simulink library "WECSim_Lib"  (R2014b)
settings: Solver=ode45  StartTime=0.0  StopTime=10.0  RelTol=1e-3
undefined symbols (not defined in the file): body, constraint, pto, simu, waves, X, Y, Z
libraries: nesl_utility x178, sm_lib x59, vrlib x12
(part 6 of 6)

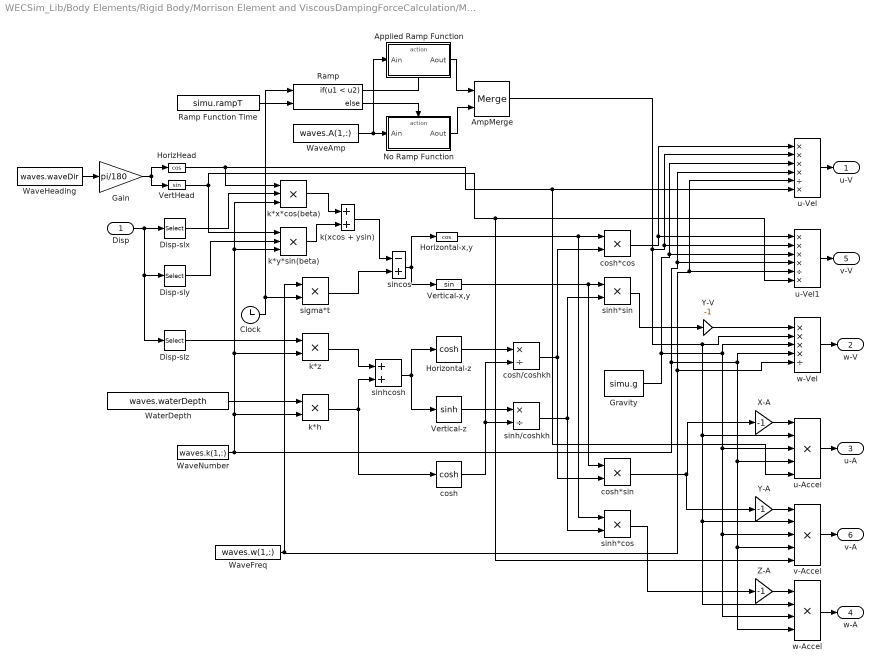
== system WECSim_Lib/Body Elements/Rigid Body/Morrison Element and ViscousDampingForceCalculation/Morrison Element Variant Subsystem/Morrison Element On/No Wave Excitation Force/MorrisonElements/OrbitalVelocity ==
  Disp : Inport
  AmpMerge : Merge
  Applied Ramp Function : Subsystem  TreatAsAtomicUnit=on
  Clock : Clock
  Disp-slx : Selector  InputPortWidth=3  Indices=[1]
  Disp-sly : Selector  InputPortWidth=3  Indices=[2]
  Disp-slz : Selector  InputPortWidth=3  Indices=[3]
  Gain : Gain  Gain=pi/180
  Gravity : Constant  Value=simu.g
  HorizHead : Trigonometry  Operator=cos
  Horizontal-x,y : Trigonometry  Operator=cos
  Horizontal-z : Trigonometry  Operator=cosh
  No Ramp Function : Subsystem  TreatAsAtomicUnit=on
  Ramp : If  NumInputs=2  IfExpression=u1 < u2
  Ramp Function Time : Constant  Value=simu.rampT
  VertHead : Trigonometry
  Vertical-x,y : Trigonometry
  Vertical-z : Trigonometry  Operator=sinh
  WaterDepth : Constant  Value=waves.waterDepth
  WaveAmp : Constant  Value=waves.A(1,:)
  WaveFreq : Constant  Value=waves.w(1,:)
  WaveHeading : Constant  Value=waves.waveDir
  WaveNumber : Constant  Value=waves.k(1,:)
  X-A : Gain  Gain=-1
  Y-A : Gain  Gain=-1
  Y-V : Gain  Gain=-1
  Z-A : Gain  Gain=-1
  cosh : Trigonometry  Operator=cosh
  cosh*cos : Product  Inputs=**
  cosh*sin : Product  Inputs=**
  cosh/coshkh : Product  Inputs=*/
  k(xcos + ysin) : Sum
  k*h : Product
  k*x*cos(beta) : Product  Inputs=3
  k*y*sin(beta) : Product  Inputs=3
  k*z : Product
  sigma*t : Product
  sincos : Sum  Inputs=-+
  sinh*cos : Product  Inputs=**
  sinh*sin : Product  Inputs=**
  sinh/coshkh : Product  Inputs=*/
  sinhcosh : Sum
  u-Accel : Product  Inputs=*****
  u-Vel : Product  Inputs=****/*
  u-Vel1 : Product  Inputs=****/*
  v-Accel : Product  Inputs=*****
  w-Accel : Product  Inputs=****
  w-Vel : Product  Inputs=****/
  u-V : Outport
  w-V : Outport  Port=2
  u-A : Outport  Port=3
  w-A : Outport  Port=4
  v-V : Outport  Port=5
  v-A : Outport  Port=6
  wires:
  Disp/1 -> Disp-slz/1, Disp-sly/1, Disp-slx/1
  WaveNumber/1 -> k*h/2, k*z/2, k*y*sin(beta)/3, k*x*cos(beta)/3, w-Vel/4, v-Accel/4, w-Accel/4, u-Accel/4, u-Vel1/4, u-Vel/4
  WaterDepth/1 -> k*h/1
  sigma*t/1 -> sincos/2
  sincos/1 -> Vertical-x,y/1, Horizontal-x,y/1
  k*z/1 -> sinhcosh/1
  k*h/1 -> cosh/1, sinhcosh/2
  sinhcosh/1 -> Vertical-z/1, Horizontal-z/1
  Horizontal-z/1 -> cosh/coshkh/1
  cosh/1 -> sinh/coshkh/2, cosh/coshkh/2
  Vertical-z/1 -> sinh/coshkh/1
  Vertical-x,y/1 -> cosh*sin/1, sinh*sin/1
  sinh/coshkh/1 -> sinh*cos/2, sinh*sin/2
  Horizontal-x,y/1 -> sinh*cos/1, cosh*cos/1
  cosh/coshkh/1 -> cosh*cos/2, cosh*sin/2
  Disp-sly/1 -> k*y*sin(beta)/2
  cosh*cos/1 -> u-Vel1/1, u-Vel/1
  AmpMerge/1 -> w-Vel/2, w-Accel/2, v-Accel/2, u-Accel/2, u-Vel1/2, u-Vel/2
  Gravity/1 -> w-Vel/3, v-Accel/3, w-Accel/3, u-Accel/3, u-Vel1/3, u-Vel/3
  sinh*sin/1 -> Y-V/1
  Y-V/1 -> w-Vel/1
  X-A/1 -> u-Accel/1
  Z-A/1 -> w-Accel/1
  w-Vel/1 -> w-V/1
  u-Accel/1 -> u-A/1
  w-Accel/1 -> w-A/1
  cosh*sin/1 -> Y-A/1, X-A/1
  sinh*cos/1 -> Z-A/1
  Ramp Function Time/1 -> Ramp/2
  Ramp/2 -> No Ramp Function/Action
  Ramp/1 -> Applied Ramp Function/Action
  Clock/1 -> Ramp/1, sigma*t/2
  No Ramp Function/1(Aout) -> AmpMerge/2
  Applied Ramp Function/1(Aout) -> AmpMerge/1
  Disp-slz/1 -> k*z/1
  WaveFreq/1 -> w-Vel/5, u-Vel1/5, u-Vel/5, sigma*t/1
  WaveAmp/1 -> Applied Ramp Function/1(Ain), No Ramp Function/1(Ain)
  WaveHeading/1 -> Gain/1
  Gain/1 -> HorizHead/1, VertHead/1
  Disp-slx/1 -> k*x*cos(beta)/2
  HorizHead/1 -> u-Accel/5, u-Vel/6, k*x*cos(beta)/1
  VertHead/1 -> k*y*sin(beta)/1, u-Vel1/6, v-Accel/5
  k*y*sin(beta)/1 -> k(xcos + ysin)/2
  k*x*cos(beta)/1 -> k(xcos + ysin)/1
  k(xcos + ysin)/1 -> sincos/1
  u-Vel1/1 -> v-V/1
  u-Vel/1 -> u-V/1
  Y-A/1 -> v-Accel/1
  v-Accel/1 -> v-A/1

== system WECSim_Lib/Body Elements/Rigid Body/Morrison Element and ViscousDampingForceCalculation/Morrison Element Variant Subsystem/Morrison Element On/No Wave Excitation Force/MorrisonElements/Rotation1 ==
  rot1 : Inport
  rot2 : Inport  Port=2
  rot3 : Inport  Port=3
  2 : Product
  3 : Product  Inputs=3
  7 : Product
  8 : Product  Inputs=3
  Combine : Concatenate  NumInputs=3  Mode=Multidimensional array  ConcatenateDimension=2
  Trigonometric Function{,1..2,6,9,11} (6 alike) : Trigonometry  Operator=cos
  Trigonometric Function{3..5,7..8,10} (6 alike) : Trigonometry
  rot11 : Product
  rot12 : Sum
  rot13 : Sum  Inputs=+-
  rot[1,1-3] : Outport
  wires:
  Trigonometric Function/1 -> rot11/1
  Trigonometric Function1/1 -> rot11/2
  rot11/1 -> Combine/1
  Trigonometric Function2/1 -> 2/1
  Trigonometric Function3/1 -> 2/2
  Trigonometric Function4/1 -> 3/1
  Trigonometric Function5/1 -> 3/2
  Trigonometric Function6/1 -> 3/3
  2/1 -> rot12/1
  3/1 -> rot12/2
  rot12/1 -> Combine/2
  Combine/1 -> rot[1,1-3]/1
  rot2/1 -> Trigonometric Function/1, Trigonometric Function5/1, Trigonometric Function10/1
  rot3/1 -> Trigonometric Function1/1, Trigonometric Function3/1, Trigonometric Function6/1, Trigonometric Function11/1, Trigonometric Function8/1
  rot1/1 -> Trigonometric Function2/1, Trigonometric Function4/1, Trigonometric Function9/1, Trigonometric Function7/1
  Trigonometric Function7/1 -> 7/1
  Trigonometric Function8/1 -> 7/2
  Trigonometric Function9/1 -> 8/1
  Trigonometric Function10/1 -> 8/2
  Trigonometric Function11/1 -> 8/3
  7/1 -> rot13/1
  8/1 -> rot13/2
  rot13/1 -> Combine/3

== system WECSim_Lib/Body Elements/Rigid Body/Morrison Element and ViscousDampingForceCalculation/Morrison Element Variant Subsystem/Morrison Element On/No Wave Excitation Force/MorrisonElements/Rotation2 ==
  rot1 : Inport
  rot2 : Inport  Port=2
  rot3 : Inport  Port=3
  2 : Product
  3 : Product  Inputs=3
  7 : Product
  8 : Product  Inputs=3
  Combine : Concatenate  NumInputs=3  Mode=Multidimensional array  ConcatenateDimension=2
  Gain : Gain  Gain=-1
  Trigonometric Function{,2..3,8..9} (5 alike) : Trigonometry  Operator=cos
  Trigonometric Function{1,4..7,10..11} (7 alike) : Trigonometry
  rot11 : Product
  rot12 : Sum  Inputs=+-
  rot13 : Sum
  rot[2,1-3] : Outport
  wires:
  Trigonometric Function/1 -> Gain/1
  Trigonometric Function1/1 -> rot11/2
  rot11/1 -> Combine/1
  Trigonometric Function2/1 -> 2/1
  Trigonometric Function3/1 -> 2/2
  Trigonometric Function4/1 -> 3/1
  Trigonometric Function5/1 -> 3/2
  Trigonometric Function6/1 -> 3/3
  2/1 -> rot12/1
  3/1 -> rot12/2
  rot12/1 -> Combine/2
  Combine/1 -> rot[2,1-3]/1
  rot2/1 -> Trigonometric Function/1, Trigonometric Function5/1, Trigonometric Function10/1
  rot3/1 -> Trigonometric Function1/1, Trigonometric Function3/1, Trigonometric Function6/1, Trigonometric Function11/1, Trigonometric Function8/1
  rot1/1 -> Trigonometric Function2/1, Trigonometric Function4/1, Trigonometric Function9/1, Trigonometric Function7/1
  Trigonometric Function7/1 -> 7/1
  Trigonometric Function8/1 -> 7/2
  Trigonometric Function9/1 -> 8/1
  Trigonometric Function10/1 -> 8/2
  Trigonometric Function11/1 -> 8/3
  7/1 -> rot13/1
  8/1 -> rot13/2
  rot13/1 -> Combine/3
  Gain/1 -> rot11/1

== system WECSim_Lib/Body Elements/Rigid Body/Morrison Element and ViscousDampingForceCalculation/Morrison Element Variant Subsystem/Morrison Element On/No Wave Excitation Force/MorrisonElements/Rotation3 ==
  rot1 : Inport
  rot2 : Inport  Port=2
  2 : Product
  7 : Product
  Combine : Concatenate  NumInputs=3  Mode=Multidimensional array  ConcatenateDimension=2
  Gain1 : Gain  Gain=-1
  TrigFun1 : Trigonometry
  TrigFun2 : Trigonometry
  TrigFun3 : Trigonometry  Operator=cos
  TrigFun4 : Trigonometry  Operator=cos
  TrigFun5 : Trigonometry  Operator=cos
  rot[3,1-3] : Outport
  wires:
  TrigFun1/1 -> Combine/1
  TrigFun3/1 -> 2/2
  2/1 -> Combine/2
  Combine/1 -> rot[3,1-3]/1
  rot2/1 -> TrigFun5/1, TrigFun3/1, TrigFun1/1
  TrigFun4/1 -> 7/1
  TrigFun5/1 -> 7/2
  rot1/1 -> TrigFun2/1, TrigFun4/1
  7/1 -> Combine/3
  TrigFun2/1 -> Gain1/1
  Gain1/1 -> 2/1

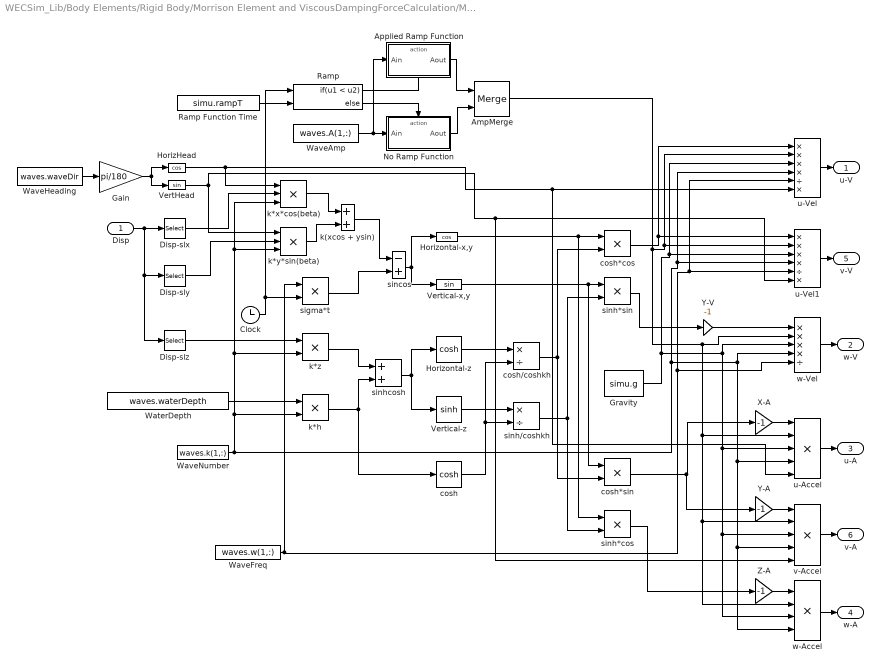
== system WECSim_Lib/Body Elements/Rigid Body/Morrison Element and ViscousDampingForceCalculation/Morrison Element Variant Subsystem/Morrison Element On/Regular Wave Excitation Force/MorrisonElements/OrbitalVelocity ==
  Disp : Inport
  AmpMerge : Merge
  Applied Ramp Function : Subsystem  TreatAsAtomicUnit=on
  Clock : Clock
  Disp-slx : Selector  InputPortWidth=3  Indices=[1]
  Disp-sly : Selector  InputPortWidth=3  Indices=[2]
  Disp-slz : Selector  InputPortWidth=3  Indices=[3]
  Gain : Gain  Gain=pi/180
  Gravity : Constant  Value=simu.g
  HorizHead : Trigonometry  Operator=cos
  Horizontal-x,y : Trigonometry  Operator=cos
  Horizontal-z : Trigonometry  Operator=cosh
  No Ramp Function : Subsystem  TreatAsAtomicUnit=on
  Ramp : If  NumInputs=2  IfExpression=u1 < u2
  Ramp Function Time : Constant  Value=simu.rampT
  VertHead : Trigonometry
  Vertical-x,y : Trigonometry
  Vertical-z : Trigonometry  Operator=sinh
  WaterDepth : Constant  Value=waves.waterDepth
  WaveAmp : Constant  Value=waves.A(1,:)
  WaveFreq : Constant  Value=waves.w(1,:)
  WaveHeading : Constant  Value=waves.waveDir
  WaveNumber : Constant  Value=waves.k(1,:)
  X-A : Gain  Gain=-1
  Y-A : Gain  Gain=-1
  Y-V : Gain  Gain=-1
  Z-A : Gain  Gain=-1
  cosh : Trigonometry  Operator=cosh
  cosh*cos : Product  Inputs=**
  cosh*sin : Product  Inputs=**
  cosh/coshkh : Product  Inputs=*/
  k(xcos + ysin) : Sum
  k*h : Product
  k*x*cos(beta) : Product  Inputs=3
  k*y*sin(beta) : Product  Inputs=3
  k*z : Product
  sigma*t : Product
  sincos : Sum  Inputs=-+
  sinh*cos : Product  Inputs=**
  sinh*sin : Product  Inputs=**
  sinh/coshkh : Product  Inputs=*/
  sinhcosh : Sum
  u-Accel : Product  Inputs=*****
  u-Vel : Product  Inputs=****/*
  u-Vel1 : Product  Inputs=****/*
  v-Accel : Product  Inputs=*****
  w-Accel : Product  Inputs=****
  w-Vel : Product  Inputs=****/
  u-V : Outport
  w-V : Outport  Port=2
  u-A : Outport  Port=3
  w-A : Outport  Port=4
  v-V : Outport  Port=5
  v-A : Outport  Port=6
  wires:
  Disp/1 -> Disp-slz/1, Disp-sly/1, Disp-slx/1
  WaveNumber/1 -> k*h/2, k*z/2, k*y*sin(beta)/3, k*x*cos(beta)/3, w-Vel/4, v-Accel/4, w-Accel/4, u-Accel/4, u-Vel1/4, u-Vel/4
  WaterDepth/1 -> k*h/1
  sigma*t/1 -> sincos/2
  sincos/1 -> Vertical-x,y/1, Horizontal-x,y/1
  k*z/1 -> sinhcosh/1
  k*h/1 -> cosh/1, sinhcosh/2
  sinhcosh/1 -> Vertical-z/1, Horizontal-z/1
  Horizontal-z/1 -> cosh/coshkh/1
  cosh/1 -> sinh/coshkh/2, cosh/coshkh/2
  Vertical-z/1 -> sinh/coshkh/1
  Vertical-x,y/1 -> cosh*sin/1, sinh*sin/1
  sinh/coshkh/1 -> sinh*cos/2, sinh*sin/2
  Horizontal-x,y/1 -> sinh*cos/1, cosh*cos/1
  cosh/coshkh/1 -> cosh*cos/2, cosh*sin/2
  Disp-sly/1 -> k*y*sin(beta)/2
  cosh*cos/1 -> u-Vel1/1, u-Vel/1
  AmpMerge/1 -> w-Vel/2, w-Accel/2, v-Accel/2, u-Accel/2, u-Vel1/2, u-Vel/2
  Gravity/1 -> w-Vel/3, v-Accel/3, w-Accel/3, u-Accel/3, u-Vel1/3, u-Vel/3
  sinh*sin/1 -> Y-V/1
  Y-V/1 -> w-Vel/1
  X-A/1 -> u-Accel/1
  Z-A/1 -> w-Accel/1
  w-Vel/1 -> w-V/1
  u-Accel/1 -> u-A/1
  w-Accel/1 -> w-A/1
  cosh*sin/1 -> Y-A/1, X-A/1
  sinh*cos/1 -> Z-A/1
  Ramp Function Time/1 -> Ramp/2
  Ramp/2 -> No Ramp Function/Action
  Ramp/1 -> Applied Ramp Function/Action
  Clock/1 -> Ramp/1, sigma*t/2
  No Ramp Function/1(Aout) -> AmpMerge/2
  Applied Ramp Function/1(Aout) -> AmpMerge/1
  Disp-slz/1 -> k*z/1
  WaveFreq/1 -> w-Vel/5, u-Vel1/5, u-Vel/5, sigma*t/1
  WaveAmp/1 -> Applied Ramp Function/1(Ain), No Ramp Function/1(Ain)
  WaveHeading/1 -> Gain/1
  Gain/1 -> HorizHead/1, VertHead/1
  Disp-slx/1 -> k*x*cos(beta)/2
  HorizHead/1 -> u-Accel/5, u-Vel/6, k*x*cos(beta)/1
  VertHead/1 -> k*y*sin(beta)/1, u-Vel1/6, v-Accel/5
  k*y*sin(beta)/1 -> k(xcos + ysin)/2
  k*x*cos(beta)/1 -> k(xcos + ysin)/1
  k(xcos + ysin)/1 -> sincos/1
  u-Vel1/1 -> v-V/1
  u-Vel/1 -> u-V/1
  Y-A/1 -> v-Accel/1
  v-Accel/1 -> v-A/1

== system WECSim_Lib/Body Elements/Rigid Body/Morrison Element and ViscousDampingForceCalculation/Morrison Element Variant Subsystem/Morrison Element On/Regular Wave Excitation Force/MorrisonElements/Rotation1 ==
  rot1 : Inport
  rot2 : Inport  Port=2
  rot3 : Inport  Port=3
  2 : Product
  3 : Product  Inputs=3
  7 : Product
  8 : Product  Inputs=3
  Combine : Concatenate  NumInputs=3  Mode=Multidimensional array  ConcatenateDimension=2
  Trigonometric Function{,1..2,6,9,11} (6 alike) : Trigonometry  Operator=cos
  Trigonometric Function{3..5,7..8,10} (6 alike) : Trigonometry
  rot11 : Product
  rot12 : Sum
  rot13 : Sum  Inputs=+-
  rot[1,1-3] : Outport
  wires:
  Trigonometric Function/1 -> rot11/1
  Trigonometric Function1/1 -> rot11/2
  rot11/1 -> Combine/1
  Trigonometric Function2/1 -> 2/1
  Trigonometric Function3/1 -> 2/2
  Trigonometric Function4/1 -> 3/1
  Trigonometric Function5/1 -> 3/2
  Trigonometric Function6/1 -> 3/3
  2/1 -> rot12/1
  3/1 -> rot12/2
  rot12/1 -> Combine/2
  Combine/1 -> rot[1,1-3]/1
  rot2/1 -> Trigonometric Function/1, Trigonometric Function5/1, Trigonometric Function10/1
  rot3/1 -> Trigonometric Function1/1, Trigonometric Function3/1, Trigonometric Function6/1, Trigonometric Function11/1, Trigonometric Function8/1
  rot1/1 -> Trigonometric Function2/1, Trigonometric Function4/1, Trigonometric Function9/1, Trigonometric Function7/1
  Trigonometric Function7/1 -> 7/1
  Trigonometric Function8/1 -> 7/2
  Trigonometric Function9/1 -> 8/1
  Trigonometric Function10/1 -> 8/2
  Trigonometric Function11/1 -> 8/3
  7/1 -> rot13/1
  8/1 -> rot13/2
  rot13/1 -> Combine/3

== system WECSim_Lib/Body Elements/Rigid Body/Morrison Element and ViscousDampingForceCalculation/Morrison Element Variant Subsystem/Morrison Element On/Regular Wave Excitation Force/MorrisonElements/Rotation2 ==
  rot1 : Inport
  rot2 : Inport  Port=2
  rot3 : Inport  Port=3
  2 : Product
  3 : Product  Inputs=3
  7 : Product
  8 : Product  Inputs=3
  Combine : Concatenate  NumInputs=3  Mode=Multidimensional array  ConcatenateDimension=2
  Gain : Gain  Gain=-1
  Trigonometric Function{,2..3,8..9} (5 alike) : Trigonometry  Operator=cos
  Trigonometric Function{1,4..7,10..11} (7 alike) : Trigonometry
  rot11 : Product
  rot12 : Sum  Inputs=+-
  rot13 : Sum
  rot[2,1-3] : Outport
  wires:
  Trigonometric Function/1 -> Gain/1
  Trigonometric Function1/1 -> rot11/2
  rot11/1 -> Combine/1
  Trigonometric Function2/1 -> 2/1
  Trigonometric Function3/1 -> 2/2
  Trigonometric Function4/1 -> 3/1
  Trigonometric Function5/1 -> 3/2
  Trigonometric Function6/1 -> 3/3
  2/1 -> rot12/1
  3/1 -> rot12/2
  rot12/1 -> Combine/2
  Combine/1 -> rot[2,1-3]/1
  rot2/1 -> Trigonometric Function/1, Trigonometric Function5/1, Trigonometric Function10/1
  rot3/1 -> Trigonometric Function1/1, Trigonometric Function3/1, Trigonometric Function6/1, Trigonometric Function11/1, Trigonometric Function8/1
  rot1/1 -> Trigonometric Function2/1, Trigonometric Function4/1, Trigonometric Function9/1, Trigonometric Function7/1
  Trigonometric Function7/1 -> 7/1
  Trigonometric Function8/1 -> 7/2
  Trigonometric Function9/1 -> 8/1
  Trigonometric Function10/1 -> 8/2
  Trigonometric Function11/1 -> 8/3
  7/1 -> rot13/1
  8/1 -> rot13/2
  rot13/1 -> Combine/3
  Gain/1 -> rot11/1

== system WECSim_Lib/Body Elements/Rigid Body/Morrison Element and ViscousDampingForceCalculation/Morrison Element Variant Subsystem/Morrison Element On/Regular Wave Excitation Force/MorrisonElements/Rotation3 ==
  rot1 : Inport
  rot2 : Inport  Port=2
  2 : Product
  7 : Product
  Combine : Concatenate  NumInputs=3  Mode=Multidimensional array  ConcatenateDimension=2
  Gain1 : Gain  Gain=-1
  TrigFun1 : Trigonometry
  TrigFun2 : Trigonometry
  TrigFun3 : Trigonometry  Operator=cos
  TrigFun4 : Trigonometry  Operator=cos
  TrigFun5 : Trigonometry  Operator=cos
  rot[3,1-3] : Outport
  wires:
  TrigFun1/1 -> Combine/1
  TrigFun3/1 -> 2/2
  2/1 -> Combine/2
  Combine/1 -> rot[3,1-3]/1
  rot2/1 -> TrigFun5/1, TrigFun3/1, TrigFun1/1
  TrigFun4/1 -> 7/1
  TrigFun5/1 -> 7/2
  rot1/1 -> TrigFun2/1, TrigFun4/1
  7/1 -> Combine/3
  TrigFun2/1 -> Gain1/1
  Gain1/1 -> 2/1

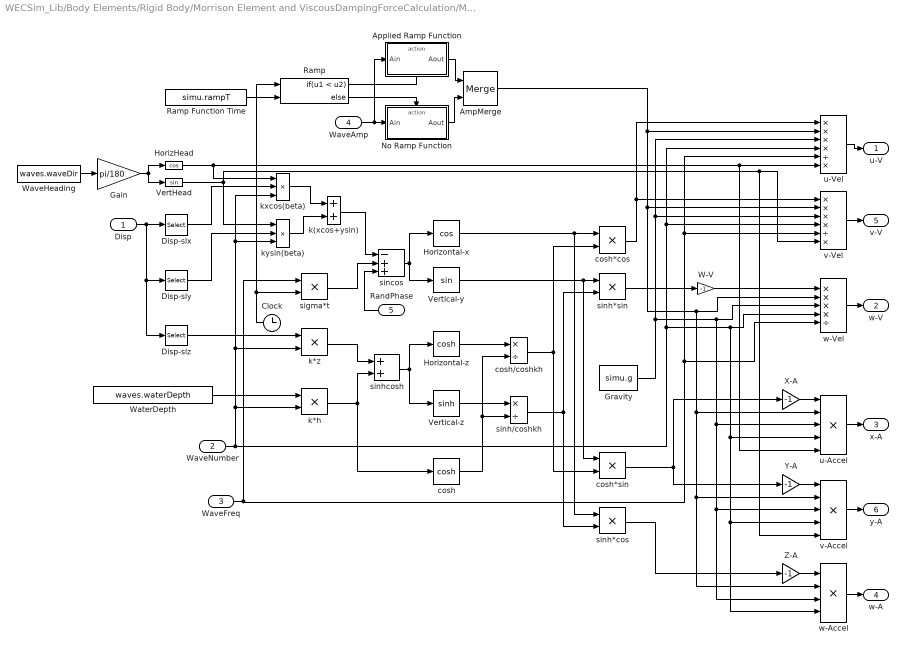
== system WECSim_Lib/Body Elements/Rigid Body/Morrison Element and ViscousDampingForceCalculation/Morrison Element Variant Subsystem/Morrison Element On/Irregular Wave Excitation Force/MorrisonElements/MorisonElementIrregular/OrbitalVelocity ==
  Disp : Inport
  WaveNumber : Inport  Port=2
  WaveFreq : Inport  Port=3
  WaveAmp : Inport  Port=4
  RandPhase : Inport  Port=5
  AmpMerge : Merge
  Applied Ramp Function : Subsystem  TreatAsAtomicUnit=on
  Clock : Clock
  Disp-slx : Selector  InputPortWidth=3  Indices=[1]
  Disp-sly : Selector  InputPortWidth=3  Indices=[2]
  Disp-slz : Selector  InputPortWidth=3  Indices=[3]
  Gain : Gain  Gain=pi/180
  Gravity : Constant  Value=simu.g
  HorizHead : Trigonometry  Operator=cos
  Horizontal-x : Trigonometry  Operator=cos
  Horizontal-z : Trigonometry  Operator=cosh
  No Ramp Function : Subsystem  TreatAsAtomicUnit=on
  Ramp : If  NumInputs=2  IfExpression=u1 < u2
  Ramp Function Time : Constant  Value=simu.rampT
  VertHead : Trigonometry
  Vertical-y : Trigonometry
  Vertical-z : Trigonometry  Operator=sinh
  W-V : Gain  Gain=-1
  WaterDepth : Constant  Value=waves.waterDepth
  WaveHeading : Constant  Value=waves.waveDir
  X-A : Gain  Gain=-1
  Y-A : Gain  Gain=-1
  Z-A : Gain  Gain=-1
  cosh : Trigonometry  Operator=cosh
  cosh*cos : Product  Inputs=**
  cosh*sin : Product  Inputs=**
  cosh/coshkh : Product  Inputs=*/
  k(xcos+ysin) : Sum
  k*h : Product
  k*z : Product
  kxcos(beta) : Product  Inputs=3
  kysin(beta) : Product  Inputs=3
  sigma*t : Product
  sincos : Sum  Inputs=-++
  sinh*cos : Product  Inputs=**
  sinh*sin : Product  Inputs=**
  sinh/coshkh : Product  Inputs=*/
  sinhcosh : Sum
  u-Accel : Product  Inputs=*****
  u-Vel : Product  Inputs=****/*
  v-Accel : Product  Inputs=*****
  v-Vel : Product  Inputs=****/*
  w-Accel : Product  Inputs=****
  w-Vel : Product  Inputs=****/
  u-V : Outport
  w-V : Outport  Port=2
  x-A : Outport  Port=3
  w-A : Outport  Port=4
  v-V : Outport  Port=5
  y-A : Outport  Port=6
  wires:
  Disp/1 -> Disp-slz/1, Disp-sly/1, Disp-slx/1
  WaveNumber/1 -> w-Vel/4, v-Accel/4, w-Accel/4, u-Accel/4, u-Vel/4, v-Vel/4, k*h/2, k*z/2, kysin(beta)/3, kxcos(beta)/3
  WaveFreq/1 -> sigma*t/1, u-Vel/5, v-Vel/5, w-Vel/5
  WaterDepth/1 -> k*h/1
  sigma*t/1 -> sincos/2
  sincos/1 -> Vertical-y/1, Horizontal-x/1
  k*z/1 -> sinhcosh/1
  k*h/1 -> cosh/1, sinhcosh/2
  sinhcosh/1 -> Vertical-z/1, Horizontal-z/1
  Horizontal-z/1 -> cosh/coshkh/1
  cosh/1 -> sinh/coshkh/2, cosh/coshkh/2
  Vertical-z/1 -> sinh/coshkh/1
  Vertical-y/1 -> sinh*sin/1, cosh*sin/1
  sinh/coshkh/1 -> sinh*cos/2, sinh*sin/2
  Horizontal-x/1 -> cosh*cos/1, sinh*cos/1
  cosh/coshkh/1 -> cosh*cos/2, cosh*sin/2
  Disp-sly/1 -> kysin(beta)/2
  cosh*cos/1 -> u-Vel/1, v-Vel/1
  AmpMerge/1 -> w-Vel/2, w-Accel/2, v-Accel/2, u-Accel/2, v-Vel/2, u-Vel/2
  sinh*sin/1 -> W-V/1
  W-V/1 -> w-Vel/1
  X-A/1 -> u-Accel/1
  Z-A/1 -> w-Accel/1
  u-Vel/1 -> u-V/1
  w-Vel/1 -> w-V/1
  u-Accel/1 -> x-A/1
  w-Accel/1 -> w-A/1
  cosh*sin/1 -> Y-A/1, X-A/1
  sinh*cos/1 -> Z-A/1
  Ramp Function Time/1 -> Ramp/2
  Ramp/2 -> No Ramp Function/Action
  Ramp/1 -> Applied Ramp Function/Action
  Clock/1 -> sigma*t/2, Ramp/1
  WaveAmp/1 -> Applied Ramp Function/1(Ain), No Ramp Function/1(Ain)
  No Ramp Function/1(Aout) -> AmpMerge/2
  Applied Ramp Function/1(Aout) -> AmpMerge/1
  Disp-slz/1 -> k*z/1
  RandPhase/1 -> sincos/3
  WaveHeading/1 -> Gain/1
  Gain/1 -> HorizHead/1, VertHead/1
  Disp-slx/1 -> kxcos(beta)/2
  HorizHead/1 -> kxcos(beta)/1, u-Vel/6, u-Accel/5
  VertHead/1 -> kysin(beta)/1, v-Accel/5, v-Vel/6
  kysin(beta)/1 -> k(xcos+ysin)/2
  kxcos(beta)/1 -> k(xcos+ysin)/1
  k(xcos+ysin)/1 -> sincos/1
  v-Vel/1 -> v-V/1
  Gravity/1 -> w-Vel/3, v-Accel/3, w-Accel/3, u-Accel/3, u-Vel/3, v-Vel/3
  Y-A/1 -> v-Accel/1
  v-Accel/1 -> y-A/1

== system WECSim_Lib/Body Elements/Rigid Body/Morrison Element and ViscousDampingForceCalculation/Morrison Element Variant Subsystem/Morrison Element On/No Wave Excitation Force/MorrisonElements/OrbitalVelocity/Applied Ramp Function ==
  Ain : Inport
  Action Port : ActionPort
  Add : Sum
  Constant : Constant  Value=2
  Constant1 : Constant
  Divide : Product  Inputs=**/
  Sine Wave : Sin  Frequency=pi/simu.rampT  Phase=pi+pi/2  SampleTime=0
  Aout : Outport
  wires:
  Ain/1 -> Divide/1
  Divide/1 -> Aout/1
  Constant/1 -> Divide/3
  Constant1/1 -> Add/1
  Sine Wave/1 -> Add/2
  Add/1 -> Divide/2

== system WECSim_Lib/Body Elements/Rigid Body/Morrison Element and ViscousDampingForceCalculation/Morrison Element Variant Subsystem/Morrison Element On/No Wave Excitation Force/MorrisonElements/OrbitalVelocity/No Ramp Function ==
  Ain : Inport
  Action Port : ActionPort
  Aout : Outport
  wires:
  Ain/1 -> Aout/1

== system WECSim_Lib/Body Elements/Rigid Body/Morrison Element and ViscousDampingForceCalculation/Morrison Element Variant Subsystem/Morrison Element On/Regular Wave Excitation Force/MorrisonElements/OrbitalVelocity/Applied Ramp Function ==
  Ain : Inport
  Action Port : ActionPort
  Add : Sum
  Constant : Constant  Value=2
  Constant1 : Constant
  Divide : Product  Inputs=**/
  Sine Wave : Sin  Frequency=pi/simu.rampT  Phase=pi+pi/2  SampleTime=0
  Aout : Outport
  wires:
  Ain/1 -> Divide/1
  Divide/1 -> Aout/1
  Constant/1 -> Divide/3
  Constant1/1 -> Add/1
  Sine Wave/1 -> Add/2
  Add/1 -> Divide/2

== system WECSim_Lib/Body Elements/Rigid Body/Morrison Element and ViscousDampingForceCalculation/Morrison Element Variant Subsystem/Morrison Element On/Regular Wave Excitation Force/MorrisonElements/OrbitalVelocity/No Ramp Function ==
  Ain : Inport
  Action Port : ActionPort
  Aout : Outport
  wires:
  Ain/1 -> Aout/1

== system WECSim_Lib/Body Elements/Rigid Body/Morrison Element and ViscousDampingForceCalculation/Morrison Element Variant Subsystem/Morrison Element On/Irregular Wave Excitation Force/MorrisonElements/MorisonElementIrregular/OrbitalVelocity/Applied Ramp Function ==
  Ain : Inport
  Action Port : ActionPort
  Add : Sum
  Constant : Constant  Value=2
  Constant1 : Constant
  Divide : Product  Inputs=**/
  Sine Wave : Sin  Frequency=pi/simu.rampT  Phase=pi+pi/2  SampleTime=0
  Aout : Outport
  wires:
  Ain/1 -> Divide/1
  Divide/1 -> Aout/1
  Constant/1 -> Divide/3
  Constant1/1 -> Add/1
  Sine Wave/1 -> Add/2
  Add/1 -> Divide/2

== system WECSim_Lib/Body Elements/Rigid Body/Morrison Element and ViscousDampingForceCalculation/Morrison Element Variant Subsystem/Morrison Element On/Irregular Wave Excitation Force/MorrisonElements/MorisonElementIrregular/OrbitalVelocity/No Ramp Function ==
  Ain : Inport
  Action Port : ActionPort
  Aout : Outport
  wires:
  Ain/1 -> Aout/1

== matlab function WECSim_Lib/Body Elements/Rigid Body/Wave Diffraction and Excitation Force Calculation/Nonlinear FK Force Variant Subsystem/With Nonlinear FroudeKrylov Force/Diffraction and Excitation Forces ==
  data: x input; elv input; center input; f output; tnorm input; area input; rho input; g input; cg input; AH input; w input; dw input; wDepth input; deepWaterWave input; k input; typeNum input; t input; phaseRand input; wp output; wpMeanFS output; dt input; dtFe input
function [f, wp, wpMeanFS]  = nonFKForce(x,elv,center,tnorm,area,rho,g,cg,AH,w,dw,wDepth,deepWaterWave,k,typeNum,t,phaseRand, dt, dtFe)
% Function to calculate buoyancy force and moment on a triangulated surface
% NOTE: This function assumes that the STL file is imported with its CG at 0,0,0

% Logic to calculate nonFKForce at reduced sample time
persistent oldForce
persistent oldWp
persistent oldWpMeanFs

if isempty(oldForce)
    [f, wp, wpMeanFS] = calc_force(x,elv,center,tnorm,area,rho,g,cg,AH,w,dw,wDepth,deepWaterWave,k,typeNum,t,phaseRand);
    oldForce = f;
    oldWp = wp;
    oldWpMeanFs = wpMeanFS;
else
    if mod(t, dtFe) < dt/2
        [f, wp, wpMeanFS] = calc_force(x,elv,center,tnorm,area,rho,g,cg,AH,w,dw,wDepth,deepWaterWave,k,typeNum,t,phaseRand);
        oldForce = f;
        oldWp = wp;
        oldWpMeanFs = wpMeanFS;
    else
        f = oldForce;
        wp = oldWp;
        wpMeanFS = oldWpMeanFs;
    end
end
end

function [f, wp, wpMeanFS]  = calc_force(x,elv,center,tnorm,area,rho,g,cg,AH,w,dw,wDepth,deepWaterWave,k,typeNum,t,phaseRand)
% Compute new tri coords after cog rotation and translation
centerMeanFS = offsetXYZ(center,cg);
avMeanFS     = tnorm .* [area area area];

% Compute new tri coords after cog rotation and translation
center = rotateXYZ(center,[1 0 0],x(4));
center = rotateXYZ(center,[0 1 0],x(5));
center = rotateXYZ(center,[0 0 1],x(6));
center = offsetXYZ(center,x);
center = offsetXYZ(center,cg);
% Compute new normal vectors coords after cog rotation and translation
tnorm = rotateXYZ(tnorm,[1 0 0],x(4));
tnorm = rotateXYZ(tnorm,[0 1 0],x(5));
tnorm = rotateXYZ(tnorm,[0 0 1],x(6));

% Copute area vectors
av = tnorm .* [area area area];

% Calculate the free surface
wpMeanFS=pDis(centerMeanFS,       0,AH,w,dw,wDepth,deepWaterWave,t,k,phaseRand,typeNum,rho,g);
wp      =pDis(center      ,     elv,AH,w,dw,wDepth,deepWaterWave,t,k,phaseRand,typeNum,rho,g);

% Calculate the hydrostatic forces
f_linear   =FK(centerMeanFS,       cg,avMeanFS,wpMeanFS);
f_nonLinear=FK(center      ,x(1:3)+cg,av      ,wp      ); 
f = f_nonLinear-f_linear;
end

function verts = offsetXYZ(verts,x)
% Function to move the position vertices
verts(:,1) = verts(:,1) + x(1);
verts(:,2) = verts(:,2) + x(2);
verts(:,3) = verts(:,3) + x(3);
end

function xn = rotateXYZ(x,ax,t)
	% function to rotate a point about an arbitrary axis
	% x: 3-componenet coordiantes
	% ax: axis about which to rotate (must be a normal vector)
	% t: rotation angle
	% xn: new coordinates after rotation
	rotMat = zeros(3);
	rotMat(1,1) = ax(1)*ax(1)*(1-cos(t))    + cos(t);
	rotMat(1,2) = ax(2)*ax(1)*(1-cos(t))    + ax(3)*sin(t);
	rotMat(1,3) = ax(3)*ax(1)*(1-cos(t))    - ax(2)*sin(t);
	rotMat(2,1) = ax(1)*ax(2)*(1-cos(t))    - ax(3)*sin(t);
	rotMat(2,2) = ax(2)*ax(2)*(1-cos(t))    + cos(t);
	rotMat(2,3) = ax(3)*ax(2)*(1-cos(t))    + ax(1)*sin(t);
	rotMat(3,1) = ax(1)*ax(3)*(1-cos(t))    + ax(2)*sin(t);
	rotMat(3,2) = ax(2)*ax(3)*(1-cos(t))    - ax(1)*sin(t);
	rotMat(3,3) = ax(3)*ax(3)*(1-cos(t))    + cos(t);
	xn = x*rotMat;
end

function f=pDis(center,elv,AH,w,dw,wDepth,deepWaterWave,t,k,phaseRand,typeNum,rho,g)
f = zeros(length(center(:,3)),1);
z=zeros(length(center(:,1)),1);
if typeNum <10
elseif typeNum <20
    f = rho.*g.*AH(1).*cos(k(1).*center(:,1)-w(1)*t);
    if deepWaterWave == 0
        z=(center(:,3)-elv).*wDepth./(wDepth+elv);
        f = f.*(cosh(k(1).*(z+wDepth))./cosh(k(1)*wDepth));
    else
        z=(center(:,3)-elv);
        f = f.*exp(k(1).*z);
    end
elseif typeNum <30
    if deepWaterWave == 0
        z=(center(:,3)-elv).*wDepth./(wDepth+elv);
        for i=1:length(AH)
            f_tmp = rho.*g.*sqrt(AH(i)*dw).*cos(k(i).*center(:,1)-w(i)*t-phaseRand(i));
            f = f + f_tmp.*(cosh(k(i).*(z+wDepth))./cosh(k(i)*wDepth));
        end
    else
        z=(center(:,3)-elv);
        for i=1:length(AH)
            f_tmp = rho.*g.*sqrt(AH(i)*dw).*cos(k(i).*center(:,1)-w(i)*t-phaseRand(i));
            f = f + f_tmp.*exp(k(i).*z);
        end
    end
end
f(z>0)=0;
end

function f = FK(center,instcg,av,wp)
% Function to calculate the force and moment about the cog due to
% hydrostatic pressure
f = zeros(6,1);

% Calculate the hydrostatic pressure at each triangle center
pressureVect = [wp wp wp].*-av;

% Compute force about cog
f(1:3) = sum(pressureVect);

% Compute moment about cog
tmp1 = ones(length(center(:,1)),1);
tmp2 = tmp1*instcg';
center2cgVec = center-tmp2;

f(4:6)= sum(cross(center2cgVec,pressureVect));
end

== matlab function WECSim_Lib/Body Elements/Rigid Body/Wave Radiation Forces Calculation/SS CI and Constant-Damping-CoeVariant Subsystem/Convolution Integral Calculation/Fluid Memory ==
  data: lenJ input; v input; F_FM output; IRKB input; CTTime input; clockTime input; numIntMidTimeSteps input
function F_FM = ConvolutionIntegral(lenJ,v,IRKB,CTTime,clockTime,numIntMidTimeSteps)

%define persistent variables
persistent velocity;
persistent kkk;
persistent oldTime;
persistent oldF_FM;

dt = CTTime(2)-CTTime(1);
len = length(CTTime);
lenJ=length(lenJ);

%update velocity
if isempty(velocity)
    kkk=0;
    velocity = zeros(lenJ,len);
    oldTime = 0;
    F_FM    = zeros(6,1);
    oldF_FM = zeros(6,1);
else
    kkk=kkk+1;
    int2=abs(kkk-floor(kkk/numIntMidTimeSteps)*numIntMidTimeSteps-1);
    if int2<0.00000001
        velocity(:,2:end) = velocity(:,1:end-1);
    end    
    if abs(clockTime-oldTime-dt)<0.00000001
        velocity(:,1) = v(:);
        %integrate
        tmpT = zeros(6,1);
        for kd=1:6
            tmpV = zeros(len,1);
            for kk=1:lenJ
                tmpY=IRKB(:,kd,kk).*velocity(kk,:)';
                tmpV = tmpV + tmpY;
            end
            tmpT(kd) = trapz(CTTime,tmpV);
        end
        F_FM=tmpT;
        oldF_FM = F_FM;
    else
        F_FM = oldF_FM;
    end
    if abs(kkk-floor(kkk/numIntMidTimeSteps)*numIntMidTimeSteps)<0.00000001; oldTime = clockTime; end     
end

end

== matlab function WECSim_Lib/Body Elements/Rigid Body/Nonlinear Wave Elevation/Linear or Instantaneous Free Surface/Instantaneous Water Free Surface  /Instantaneous FS ==
  data: x input; center input; f output; cg input; AH input; w input; dw input; k input; typeNum input; t input; rampT input; phaseRand input; waveDir input; dt input; dtFe input
function f  = waveElevation(x,center,cg,AH,w,dw,k,typeNum,t,rampT,phaseRand,waveDir, dt, dtFe)
% Function to calculate buoyancy force and moment on a triangulated surface
% NOTE: This function assumes that the STL file is imported with its CG at 0,0,0

persistent oldElev

if isempty(oldElev)
    f = calc_elev(x,center,cg,AH,w,dw,k,typeNum,t,rampT,phaseRand, waveDir);
    oldElev = f;
else
    if mod(t, dtFe) < dt/2
        f = calc_elev(x,center,cg,AH,w,dw,k,typeNum,t,rampT,phaseRand, waveDir);
        oldElev = f;
    else
        f = oldElev;
    end
end
end


function f = calc_elev(x,center,cg,AH,w,dw,k,typeNum,t,rampT,phaseRand,waveDir)
% Compute new tri center coords after cog rotation and translation
center = rotateXYZ(center,[1 0 0],x(4));
center = rotateXYZ(center,[0 1 0],x(5));
center = rotateXYZ(center,[0 0 1],x(6));
center = offsetXYZ(center,x);
center = offsetXYZ(center,cg);

% Calculate the free surface
f=waveElev(center,AH,w,dw,t,k,rampT,phaseRand,typeNum,waveDir);

end

function verts = offsetXYZ(verts,x)
% Function to move the position vertices
verts(:,1) = verts(:,1) + x(1);
verts(:,2) = verts(:,2) + x(2);
verts(:,3) = verts(:,3) + x(3);
end

function xn = rotateXYZ(x,ax,t)
	% function to rotate a point about an arbitrary axis
	% x: 3-componenet coordiantes
	% ax: axis about which to rotate (must be a normal vector)
	% t: rotation angle
	% xn: new coordinates after rotation
	rotMat = zeros(3);
	rotMat(1,1) = ax(1)*ax(1)*(1-cos(t))    + cos(t);
	rotMat(1,2) = ax(2)*ax(1)*(1-cos(t))    + ax(3)*sin(t);
	rotMat(1,3) = ax(3)*ax(1)*(1-cos(t))    - ax(2)*sin(t);
	rotMat(2,1) = ax(1)*ax(2)*(1-cos(t))    - ax(3)*sin(t);
	rotMat(2,2) = ax(2)*ax(2)*(1-cos(t))    + cos(t);
	rotMat(2,3) = ax(3)*ax(2)*(1-cos(t))    + ax(1)*sin(t);
	rotMat(3,1) = ax(1)*ax(3)*(1-cos(t))    + ax(2)*sin(t);
	rotMat(3,2) = ax(2)*ax(3)*(1-cos(t))    - ax(1)*sin(t);
	rotMat(3,3) = ax(3)*ax(3)*(1-cos(t))    + cos(t);
	xn = x*rotMat;
end

function f=waveElev(center,AH,w,dw,t,k,rampT,phaseRand,typeNum,waveDir)
f = zeros(length(center(:,3)),1);
cx = center(:,1);
cy = center(:,2);
X = cx*cos(waveDir*pi/180) + cy*sin(waveDir*pi/180);
if typeNum <10
elseif typeNum <20
    f = AH(1).*cos(k(1).*X-w(1)*t);
elseif typeNum <30
    tmp=sqrt(AH.*dw);
    tmp1 = ones(1,length(center(:,1)));
    tmp2 = (w.*t+phaseRand)*tmp1;
    tmp3 = cos(k*X'- tmp2);
    f(:,1) = tmp3'*tmp;
end
if t<=rampT
    rampF = (1+cos(pi+pi*t/rampT))/2;
    f = f.*rampF;
end

end

== matlab function WECSim_Lib/Body Elements/Rigid Body/Hydrostatic Restoring Force Calculation/Linear and Nonlinear Restoring Force Variant Subsystem/Nonlinear Hydrostatic Restoring Force/Diffarction and Excitation Forces1 ==
  data: x input; elv input; center input; f output; tnorm input; area input; rho input; g input; cg input; p output; dt input; dtFe input; t input
function [f,p]  = nonLinearBuoyancy(x,elv,center,tnorm,area,rho,g,cg,dt,dtFe,t)
% Function to calculate buoyancy force and moment on a triangulated surface
% NOTE: This function assumes that the STL file is imported with its CG at 0,0,0
persistent oldF 
persistent oldP

if isempty(oldF)
    [f,p] = calc_buoyancy(x,elv,center,tnorm,area,rho,g,cg);
    oldF  = f;
    oldP  = p;
else
    if mod(t, dtFe) < dt/2
        [f,p] = calc_buoyancy(x,elv,center,tnorm,area,rho,g,cg);
        oldF  = f;
        oldP  = p;
    else
        f  = oldF;
        p  = oldP;
    end
end
end


function [f,p] = calc_buoyancy(x,elv,center,tnorm,area,rho,g,cg)
% Compute new tri coords after cog rotation and translation
center = rotateXYZ(center,[1 0 0],x(4));
center = rotateXYZ(center,[0 1 0],x(5));
center = rotateXYZ(center,[0 0 1],x(6));
center = offsetXYZ(center,x);
center = offsetXYZ(center,cg);
% Compute new normal vectors coords after cog rotation
tnorm = rotateXYZ(tnorm,[1 0 0],x(4));
tnorm = rotateXYZ(tnorm,[0 1 0],x(5));
tnorm = rotateXYZ(tnorm,[0 0 1],x(6));

% Calculate the hydrostatic forces
av = tnorm .* [area area area];
[f,p]=fHydrostatic(center,elv,x(1:3)+cg,av,rho,g); 
end

function verts = offsetXYZ(verts,x)
% Function to move the position vertices
verts(:,1) = verts(:,1) + x(1);
verts(:,2) = verts(:,2) + x(2);
verts(:,3) = verts(:,3) + x(3);
end

function xn = rotateXYZ(x,ax,t)
	% function to rotate a point about an arbitrary axis
	% x: 3-componenet coordiantes
	% ax: axis about which to rotate (must be a normal vector)
	% t: rotation angle
	% xn: new coordinates after rotation
	rotMat = zeros(3);
	rotMat(1,1) = ax(1)*ax(1)*(1-cos(t))    + cos(t);
	rotMat(1,2) = ax(2)*ax(1)*(1-cos(t))    + ax(3)*sin(t);
	rotMat(1,3) = ax(3)*ax(1)*(1-cos(t))    - ax(2)*sin(t);
	rotMat(2,1) = ax(1)*ax(2)*(1-cos(t))    - ax(3)*sin(t);
	rotMat(2,2) = ax(2)*ax(2)*(1-cos(t))    + cos(t);
	rotMat(2,3) = ax(3)*ax(2)*(1-cos(t))    + ax(1)*sin(t);
	rotMat(3,1) = ax(1)*ax(3)*(1-cos(t))    + ax(2)*sin(t);
	rotMat(3,2) = ax(2)*ax(3)*(1-cos(t))    - ax(1)*sin(t);
	rotMat(3,3) = ax(3)*ax(3)*(1-cos(t))    + cos(t);
	xn = x*rotMat;
end

function [f,p] = fHydrostatic(center,elv,instcg,av,rho,g)
% Function to calculate the force and moment about the cog due to
% hydrostatic pressure
f = zeros(6,1);

% Zeor out regions above the mean free surface
z=center(:,3); z((z-elv)>0)=0;

% Calculate the hydrostatic pressure at each triangle center
pressureVect = rho*g.*[-z -z -z].*-av;
p = rho*g.*-z;
% Compute force about cog
f(1:3) = sum(pressureVect);

tmp1 = ones(length(center(:,1)),1);
tmp2 = tmp1*instcg';
center2cgVec = center-tmp2;

f(4:6)= sum(cross(center2cgVec,pressureVect));
end

== matlab function WECSim_Lib/Constraints/Floating (6DOF)/Mooring/MoorDyn/MoorDyn/Triggered Subsystem/MATLAB Function ==
  data: X input; FLines output; XD input; Time input; CoupTime input
function FLines  = MoorDyn_matlab_FCN(X,XD,Time,CoupTime)

    FLines = zeros(1,6);
    coder.extrinsic('MoorDyn_caller');
    
    FLines = MoorDyn_caller(X,XD,Time-CoupTime,CoupTime);

== matlab function WECSim_Lib/Constraints/Floating (3DOF)/Mooring/MoorDyn/MoorDyn/Triggered Subsystem/MATLAB Function ==
  data: X input; FLines output; XD input; Time input; CoupTime input
function FLines  = MoorDyn_matlab_FCN(X,XD,Time,CoupTime)

    FLines = zeros(1,6);
    coder.extrinsic('MoorDyn_caller');
    
    FLines = MoorDyn_caller(X,XD,Time-CoupTime,CoupTime);

== matlab function WECSim_Lib/Constraints/Heave/Mooring/MoorDyn/MoorDyn/Triggered Subsystem/MATLAB Function ==
  data: X input; FLines output; XD input; Time input; CoupTime input
function FLines  = MoorDyn_matlab_FCN(X,XD,Time,CoupTime)

    FLines = zeros(1,6);
    coder.extrinsic('MoorDyn_caller');
    
    FLines = MoorDyn_caller(X,XD,Time-CoupTime,CoupTime);

== matlab function WECSim_Lib/Body Elements/Rigid Body/Structure/Motion Sensor/Angle ==
  data: Q input; E output
function E  = EulerAngle(Q)
%#codegen
E=zeros(3,1);
E(1) = atan2( (2*(Q(1)*Q(2)+Q(3)*Q(4))), (1-2* (Q(2)^2+Q(3)^2) ) );
E(2) = asin( 2* (Q(1)*Q(3) - Q(4)*Q(2)));
E(3) = atan2( (2*(Q(1)*Q(4)+Q(2)*Q(3))), (1-2* (Q(3)^2+Q(4)^2) ) );

== matlab function WECSim_Lib/Constraints/Pitch/Mooring/MoorDyn/MoorDyn/Triggered Subsystem/MATLAB Function ==
  data: X input; FLines output; XD input; Time input; CoupTime input
function FLines  = MoorDyn_matlab_FCN(X,XD,Time,CoupTime)

    FLines = zeros(1,6);
    coder.extrinsic('MoorDyn_caller');
    
    FLines = MoorDyn_caller(X,XD,Time-CoupTime,CoupTime);

== matlab function WECSim_Lib/Constraints/Surge/Mooring/MoorDyn/MoorDyn/Triggered Subsystem/MATLAB Function ==
  data: X input; FLines output; XD input; Time input; CoupTime input
function FLines  = MoorDyn_matlab_FCN(X,XD,Time,CoupTime)

    FLines = zeros(1,6);
    coder.extrinsic('MoorDyn_caller');
    
    FLines = MoorDyn_caller(X,XD,Time-CoupTime,CoupTime);
